simulink library "LopesDevelopmentLibrary"  (R2015b)
settings: Solver=ode45  StartTime=0.0  StopTime=10.0  RelTol=1e-3
values from neighbouring files (symbols this model uses):
  d2r = @(d) d*(pi/180)    [LopesDevelopmentLibrary_LoadParameters.m]
  ts = LopesParams.ts    [LopesDevelopmentLibrary_LoadParameters.m]
undefined symbols (not defined in the file or in its folder): anyParameterChanged, DiscIntNeverNeededParam, gcbh, LHF, LKF, LopesParams, macaddr, mxpcnetworkconfig, mxpcrtudprx, mxpcrtudptx, patientParametersChanged, port, PX, PZ, RHF, RKF, SelectorLOPESInSize, StrideTime_s, Time
undefined symbols (not defined in the file): LopesParamsSendDataArrayLen
libraries: LopesDevelopmentLibrary x288, simulink x98, dspmtrx3 x47, xpciplib x6, xpcnetworkbufferlib x5, dspsigops x4, dspstat3 x3, xpcethernetlib x2, visionstatistics x2, xpcseriallib x2, nmc x1, simulink_extras x1
(part 10 of 12)

== system LopesDevelopmentLibrary/Mindwalker/Mindwalker_Lopes_Conversion/VisualizeStickFigure/Subsystem ==
  In1 : Inport
  Enable : EnablePort
  Interpreted MATLAB Function : MATLABFcn  MATLABFcn=Mindwalker_ShowStickFigure  OutputDimensions=0
  wires:
  In1/1 -> Interpreted MATLAB Function/1

== system LopesDevelopmentLibrary/Robot control blocks/FromLopes/ParseString/MeasuredSegmentToAnatomicAngles ==
  note: This block works for angles, angular velocities and accelerations as well.
  note: Order of the signals:
      | PX (forward)
      | PZ (right)
      | LHA (Left hip abduction)
      | LHF (Left hip flexion)
      | LKF (Left knee flexion)
      | RHA
      | RHF
      | RKF
      |
      | PY (up)
      | PAX (Pelvis axial rotation (right hip forward=positive?)
      | POB (Pelvis obliquity (left hip up =positive)
  segmentModelX : Inport
  Demux3 : Demux  Outputs=15
  MinusRHA : UnaryMinus
  Mux : Mux  Inputs=11
  SubtractKLF : Sum  Inputs=+-
  SubtractRKF : Sum  Inputs=+-
  Terminator{1..4} (4 alike) : Terminator
  Anatomic : Outport
  wires:
  Demux3/14 -> Terminator2/1  "LAE"
  Demux3/13 -> Mux/11  "POB"
  Demux3/12 -> Mux/10  "PAX"
  Demux3/11 -> Mux/9  "PY"
  Demux3/15 -> Terminator1/1  "RAE"
  Mux/1 -> Anatomic/1
  Demux3/7 -> MinusRHA/1  "RHA"
  segmentModelX/1 -> Demux3/1
  SubtractRKF/1 -> Mux/8  "RKF"
  Demux3/8 -> Mux/7, SubtractRKF/1  "RHF"
  MinusRHA/1 -> Mux/6  "RHA"
  SubtractKLF/1 -> Mux/5  "LKF"
  Demux3/4 -> Mux/4, SubtractKLF/1  "LHF"
  Demux3/3 -> Mux/3  "LHA"
  Demux3/2 -> Mux/2  "PZ"
  Demux3/1 -> Mux/1  "PX"
  Demux3/5 -> SubtractKLF/2  "RHA"
  Demux3/6 -> Terminator4/1  "RHF"
  Demux3/9 -> SubtractRKF/2  "RHF"
  Demux3/10 -> Terminator3/1

== system LopesDevelopmentLibrary/Robot control blocks/FromLopes/ParseString/MeasuredSegmentToAnatomicAngles1 ==
  note: Order of the signals:
      | PX (forward)
      | PZ (right)
      | LHA (Left hip abduction)
      | LHF (Left hip flexion)
      | LKF (Left knee flexion)
      | RHA
      | RHF
      | RKF
      |
      | PY (up)
      | PAX (Pelvis axial rotation (right hip forward=positive?)
      | POB (Pelvis obliquity (left hip up =positive)
  note: This block works for angles, angular velocities and accelerations as well.
  segmentModelX : Inport
  Demux3 : Demux  Outputs=15
  MinusRHA : UnaryMinus
  Mux : Mux  Inputs=11
  SubtractKLF : Sum  Inputs=+-
  SubtractRKF : Sum  Inputs=+-
  Terminator{1..4} (4 alike) : Terminator
  Anatomic : Outport
  wires:
  Demux3/10 -> Terminator3/1
  Demux3/9 -> SubtractRKF/2  "RHF"
  Demux3/6 -> Terminator4/1  "RHF"
  Demux3/5 -> SubtractKLF/2  "RHA"
  Demux3/1 -> Mux/1  "PX"
  Demux3/2 -> Mux/2  "PZ"
  Demux3/3 -> Mux/3  "LHA"
  Demux3/4 -> SubtractKLF/1, Mux/4  "LHF"
  SubtractKLF/1 -> Mux/5  "LKF"
  MinusRHA/1 -> Mux/6  "RHA"
  Demux3/8 -> SubtractRKF/1, Mux/7  "RHF"
  SubtractRKF/1 -> Mux/8  "RKF"
  segmentModelX/1 -> Demux3/1
  Demux3/7 -> MinusRHA/1  "RHA"
  Mux/1 -> Anatomic/1
  Demux3/15 -> Terminator1/1  "RAE"
  Demux3/11 -> Mux/9  "PY"
  Demux3/12 -> Mux/10  "PAX"
  Demux3/13 -> Mux/11  "POB"
  Demux3/14 -> Terminator2/1  "LAE"

== system LopesDevelopmentLibrary/Robot control blocks/FromLopes/ParseString/MeasuredSegmentToAnatomicAngles2 ==
  note: This block works for angles, angular velocities and accelerations as well.
  note: Order of the signals:
      | PX (forward)
      | PZ (right)
      | LHA (Left hip abduction)
      | LHF (Left hip flexion)
      | LKF (Left knee flexion)
      | RHA
      | RHF
      | RKF
      |
      | PY (up)
      | PAX (Pelvis axial rotation (right hip forward=positive?)
      | POB (Pelvis obliquity (left hip up =positive)
  segmentModelX : Inport
  Demux3 : Demux  Outputs=15
  MinusRHA : UnaryMinus
  Mux : Mux  Inputs=11
  SubtractKLF : Sum  Inputs=+-
  SubtractRKF : Sum  Inputs=+-
  Terminator{1..4} (4 alike) : Terminator
  Anatomic : Outport
  wires:
  Demux3/14 -> Terminator2/1  "LAE"
  Demux3/13 -> Mux/11  "POB"
  Demux3/12 -> Mux/10  "PAX"
  Demux3/11 -> Mux/9  "PY"
  Demux3/15 -> Terminator1/1  "RAE"
  Mux/1 -> Anatomic/1
  Demux3/7 -> MinusRHA/1  "RHA"
  segmentModelX/1 -> Demux3/1
  SubtractRKF/1 -> Mux/8  "RKF"
  Demux3/8 -> Mux/7, SubtractRKF/1  "RHF"
  MinusRHA/1 -> Mux/6  "RHA"
  SubtractKLF/1 -> Mux/5  "LKF"
  Demux3/4 -> Mux/4, SubtractKLF/1  "LHF"
  Demux3/3 -> Mux/3  "LHA"
  Demux3/2 -> Mux/2  "PZ"
  Demux3/1 -> Mux/1  "PX"
  Demux3/5 -> SubtractKLF/2  "RHA"
  Demux3/6 -> Terminator4/1  "RHF"
  Demux3/9 -> SubtractRKF/2  "RHF"
  Demux3/10 -> Terminator3/1

== system LopesDevelopmentLibrary/Robot control blocks/FromLopes/ParseString/MeasuredSegmentToAnatomicAngles3 ==
  note: Order of the signals:
      | PX (forward)
      | PZ (right)
      | LHA (Left hip abduction)
      | LHF (Left hip flexion)
      | LKF (Left knee flexion)
      | RHA
      | RHF
      | RKF
      |
      | PY (up)
      | PAX (Pelvis axial rotation (right hip forward=positive?)
      | POB (Pelvis obliquity (left hip up =positive)
  note: This block works for angles, angular velocities and accelerations as well.
  segmentModelX : Inport
  Demux3 : Demux  Outputs=15
  MinusRHA : UnaryMinus
  Mux : Mux  Inputs=11
  SubtractKLF : Sum  Inputs=+-
  SubtractRKF : Sum  Inputs=+-
  Terminator{1..4} (4 alike) : Terminator
  Anatomic : Outport
  wires:
  Demux3/10 -> Terminator3/1
  Demux3/9 -> SubtractRKF/2  "RHF"
  Demux3/6 -> Terminator4/1  "RHF"
  Demux3/5 -> SubtractKLF/2  "RHA"
  Demux3/1 -> Mux/1  "PX"
  Demux3/2 -> Mux/2  "PZ"
  Demux3/3 -> Mux/3  "LHA"
  Demux3/4 -> SubtractKLF/1, Mux/4  "LHF"
  SubtractKLF/1 -> Mux/5  "LKF"
  MinusRHA/1 -> Mux/6  "RHA"
  Demux3/8 -> SubtractRKF/1, Mux/7  "RHF"
  SubtractRKF/1 -> Mux/8  "RKF"
  segmentModelX/1 -> Demux3/1
  Demux3/7 -> MinusRHA/1  "RHA"
  Mux/1 -> Anatomic/1
  Demux3/15 -> Terminator1/1  "RAE"
  Demux3/11 -> Mux/9  "PY"
  Demux3/12 -> Mux/10  "PAX"
  Demux3/13 -> Mux/11  "POB"
  Demux3/14 -> Terminator2/1  "LAE"

== system LopesDevelopmentLibrary/Robot control blocks/FromLopes/ParseString/MeasuredSegmentToAnatomicForce ==
  note: We can (at this moment) only get the joint forces of the patient
      | in absolute torques, i.e. torques on the limbs instead of joint torques. In order to
      | convert this to (relative) anatomical torques, we need this block.
      | This block works for forces/torques only (it does the inverse transformation
      | of the MeasuredSegmentToAnatomicVelocity block).
  segmentMeasForce : Inport
  AddLHF : Sum
  AddRHF : Sum
  Demux3 : Demux  Outputs=10
  MinusLKF : UnaryMinus
  MinusRHA : UnaryMinus
  MinusRKF : UnaryMinus
  Mux : Mux  Inputs=8
  Terminator : Terminator
  Terminator1 : Terminator
  AnatomicForce : Outport
  wires:
  Demux3/6 -> Terminator1/1  "RHF"
  Demux3/8 -> AddRHF/1  "RHF"
  Mux/1 -> AnatomicForce/1
  Demux3/7 -> MinusRHA/1  "RHA"
  MinusRKF/1 -> Mux/8  "RKF"
  AddRHF/1 -> Mux/7  "RHF"
  MinusRHA/1 -> Mux/6  "RHA"
  AddLHF/1 -> Mux/4  "LHF"
  Demux3/3 -> Mux/3  "LHA"
  Demux3/2 -> Mux/2  "PZ"
  Demux3/1 -> Mux/1  "PX"
  Demux3/9 -> AddRHF/2, MinusRKF/1  "RHF"
  Demux3/10 -> Terminator/1
  Demux3/4 -> AddLHF/1  "LHF"
  Demux3/5 -> AddLHF/2, MinusLKF/1  "RHA"
  MinusLKF/1 -> Mux/5  "LKF"
  segmentMeasForce/1 -> Demux3/1

== system LopesDevelopmentLibrary/Robot control blocks/FromLopes/ParseString/Vector2CartesianPositionsBus ==
  note: Output:
      | Cartesian positions (i.e., 3-element vectors) of:
      | Pelvis
      | LeftHip
      | LeftKnee
      | LeftAnkle
      | RightHip
      | RightKnee
      | RightAnkle
      |
      | Each vector: [X,Y, Z] = [Forward, Up, Right]
  In : Inport
  Demux3 : Demux  Outputs=11
  Mux : Mux  Inputs=7
  Terminator{1..4} (4 alike) : Terminator
  CartesianPositions : Outport
  wires:
  Demux3/9 -> Mux/7  "pRightAnkle"
  Demux3/4 -> Mux/4  "pLeftAnkle"
  Demux3/1 -> Mux/1  "pPelvis"
  Demux3/2 -> Mux/2  "pLeftHip"
  Demux3/3 -> Mux/3  "pLeftKnee"
  Demux3/5 -> Terminator1/1  "pLeftHeel"
  Demux3/6 -> Terminator4/1  "pLeftToe"
  Demux3/7 -> Mux/5  "pRightHip"
  Demux3/8 -> Mux/6  "pRightKnee"
  Demux3/10 -> Terminator2/1  "pRightHeel"
  Demux3/11 -> Terminator3/1  "pRightToe"
  In/1 -> Demux3/1
  Mux/1 -> CartesianPositions/1

== system LopesDevelopmentLibrary/Robot control blocks/FromLopes/ParseString/~Debug ==

== system LopesDevelopmentLibrary/Robot control blocks/ToLopes/GenerateVelocities/UseNumericalDerivative ==
  Positions : Inport
  Enable : EnablePort
  Discrete Derivative : simulink/Discrete/Discrete Derivative  gainval=1.0  ICPrevScaledInput=0.0  InputProcessing=Inherited  OutMin=[]  OutMax=[]  OutDataType=fixdt(1, 16)  OutScaling=2^-10  DoSatur=off
  Gain : Gain
  Velocities : Outport
  wires:
  Positions/1 -> Discrete Derivative/1
  Discrete Derivative/1 -> Gain/1
  Gain/1 -> Velocities/1

== system LopesDevelopmentLibrary/Robot control blocks/ToLopes/GenerateVelocities/UseNumericalDerivativeFiltered ==
  Positions : Inport
  Enable : EnablePort
  FirstOrderLowPassFilter : Subsystem  mask{Tau=0.01}
  Gain : Gain
  Velocities : Outport
  wires:
  FirstOrderLowPassFilter/1(ddt) -> Gain/1
  Positions/1 -> FirstOrderLowPassFilter/1(In)
  Gain/1 -> Velocities/1

== system LopesDevelopmentLibrary/Robot control blocks/ToLopes/GenerateVelocities/UseUserVelocity ==
  Velocities_in : Inport
  Enable : EnablePort
  Gain : Gain  Gain=ones(1,8)
  Velocities : Outport
  wires:
  Velocities_in/1 -> Gain/1
  Gain/1 -> Velocities/1

== system LopesDevelopmentLibrary/Robot control blocks/ToLopes/GenerateVelocities/UseZeros ==
  Enable : EnablePort
  Constant : Constant  Value=[0,0,0,0,0,0,0,0]
  Velocities : Outport  InitialOutput=[0,0,0,0,0,0,0,0]
  wires:
  Constant/1 -> Velocities/1

== system LopesDevelopmentLibrary/Robot control blocks/ToLopes/SwitchVelocitiesOnly/UseAnalyticalVelocityOnly ==
  ModelPosIn : Inport
  DesSprPos : Inport  Port=2
  DesSprVel : Inport  Port=3
  Enable : EnablePort
  Add : Sum  Inputs=-+
  Add1 : Sum
  Constant : Constant  Value=0  OutDataTypeStr=boolean
  Constant1 : Constant  Value=[0,0,0,0,0,0,0,0]
  OneOverTau_s : Gain
  UpdateSpringPos : Outport  InitialOutput=[false]
  SpringPositions : Outport  Port=2  InitialOutput=[0,0,0,0,0,0,0,0]
  SpringVelocities : Outport  Port=3  InitialOutput=[0,0,0,0,0,0,0,0]
  wires:
  Constant1/1 -> SpringPositions/1
  Constant/1 -> UpdateSpringPos/1
  Add1/1 -> SpringVelocities/1
  Add/1 -> OneOverTau_s/1
  OneOverTau_s/1 -> Add1/1
  DesSprVel/1 -> Add1/2
  DesSprPos/1 -> Add/2
  ModelPosIn/1 -> Add/1

== system LopesDevelopmentLibrary/Robot control blocks/ToLopes/SwitchVelocitiesOnly/UsePositionsAndVelocities ==
  DesSprPos : Inport
  DesSprVel : Inport  Port=2
  Enable : EnablePort
  Constant : Constant  Value=true  OutDataTypeStr=boolean
  UpdateSpringPos : Outport  InitialOutput=[false]
  SpringPositions : Outport  Port=2  InitialOutput=[0,0,0,0,0,0,0,0]
  SpringVelocities : Outport  Port=3  InitialOutput=[0,0,0,0,0,0,0,0]
  wires:
  Constant/1 -> UpdateSpringPos/1
  DesSprVel/1 -> SpringVelocities/1
  DesSprPos/1 -> SpringPositions/1

== system LopesDevelopmentLibrary/BlocksForInternalUse/LLC Communication/LLC Network Configuration/Variant Network Init/Init_NonRT_UDP ==
  note: No initialization needed for Non RT UDP.
  Dummy_in : Inport
  Dummy1 : Terminator
  Dummy2 : Constant
  Dummy_out : Outport
  wires:
  Dummy_in/1 -> Dummy1/1
  Dummy2/1 -> Dummy_out/1

== system LopesDevelopmentLibrary/BlocksForInternalUse/LLC Communication/LLC Network Configuration/Variant Network Init/Init_RT_2012b ==
  Dummy_in : Inport
  Dummy1 : Terminator
  Dummy2 : Constant
  "Network Configuration_RT_2012b " : LopesDevelopmentLibrary/BlocksForInternalUse/LLC Communication/UDP_Blocks/Network Configuration_RT_2012b   IpAddress=LopesParams.Communication.ipSelf_RT  SubnetMask=255.255.255.0  Gateway=0.0.0.0  EthDrv=Intel Gigabit  PciBus=LopesParams.Communication.busSelf_RT  PciSlot=LopesParams.Communication.slotSelf_RT
  Dummy_out : Outport
  wires:
  Dummy2/1 -> Dummy_out/1
  Dummy_in/1 -> Dummy1/1

== system LopesDevelopmentLibrary/BlocksForInternalUse/LLC Communication/LLC Network Configuration/Variant Network Init/Init_RT_2014b ==
  Dummy_in : Inport
  Dummy2 : Constant
  Dummy3 : Terminator
  "Network Configuration_RT_2014b " : LopesDevelopmentLibrary/BlocksForInternalUse/LLC Communication/UDP_Blocks/Network Configuration_RT_2014b   ID=1  IpAddress=LopesParams.Communication.ipSelf_RT  SubnetMask=255.255.255.0  Gateway=0.0.0.0  EthDrv=Intel Gigabit  PciBus=LopesParams.Communication.busSelf_RT  PciSlot=LopesParams.Communication.slotSelf_RT  udpID=0
  Dummy_out : Outport
  wires:
  Dummy_in/1 -> Dummy3/1
  Dummy2/1 -> Dummy_out/1

== system LopesDevelopmentLibrary/BlocksForInternalUse/LLC Communication/LLC Network Configuration/Variant Network Init/Init_RT_2015b ==
  Dummy_in : Inport
  Dummy2 : Constant
  Dummy3 : Terminator
  Network Configuration_RT_2015b : LopesDevelopmentLibrary/BlocksForInternalUse/LLC Communication/UDP_Blocks/Network Configuration_RT_2015b  ID=1  IpAddress=LopesParams.Communication.ipSelf_RT  SubnetMask=255.255.255.0  Gateway=0.0.0.0  EthDrv=Intel Gigabit  PciBus=LopesParams.Communication.busSelf_RT  PciSlot=LopesParams.Communication.slotSelf_RT  udpID=0  MulticastList=[]  Multicast={}
  Dummy_out : Outport
  wires:
  Dummy2/1 -> Dummy_out/1
  Dummy_in/1 -> Dummy3/1

== system LopesDevelopmentLibrary/BlocksForInternalUse/LLC Communication/LLCReceiveUDP/UDPReceiveVariantChannel/Receive_Non_RT ==
  Dummy_in : Inport
  Receive_Non-RT : LopesDevelopmentLibrary/BlocksForInternalUse/LLC Communication/UDP_Blocks/Receive_Non-RT  ipAddress='0.0.0.0'  ipPort=port  width=1500  vblLen=on  sampletime=LopesParams.ts
  Terminator : Terminator
  RecvData : Outport
  RecvLen : Outport  Port=2
  wires:
  Receive_Non-RT/2 -> RecvLen/1
  Receive_Non-RT/1 -> RecvData/1
  Dummy_in/1 -> Terminator/1

== system LopesDevelopmentLibrary/BlocksForInternalUse/LLC Communication/LLCReceiveUDP/UDPReceiveVariantChannel/Receive_RT_2015b ==
  Dummy_in : Inport
  Receive_RT_2015b : LopesDevelopmentLibrary/BlocksForInternalUse/LLC Communication/UDP_Blocks/Receive_RT_2015b  ID=1  Receive1='0.0.0.0'  Receive2=port  Receive3=1500  Receive4=LopesParams.ts  udpID=0
  Terminator : Terminator
  RecvData : Outport
  RecvLen : Outport  Port=2
  wires:
  Dummy_in/1 -> Terminator/1
  Receive_RT_2015b/1 -> RecvData/1
  Receive_RT_2015b/2 -> RecvLen/1

== system LopesDevelopmentLibrary/BlocksForInternalUse/LLC Communication/LLCReceiveUDP/UDPReceiveVariantChannel/Receive_RT_R2012b ==
  Dummy_in : Inport
  "Receive_RT_2012b " : LopesDevelopmentLibrary/BlocksForInternalUse/LLC Communication/UDP_Blocks/Receive_RT_2012b   Receive1='0.0.0.0'  Receive2=port  Receive3=1500  Receive4=LopesParams.ts
  Terminator : Terminator
  RecvData : Outport
  RecvLen : Outport  Port=2
  wires:
  "Receive_RT_2012b "/1 -> RecvData/1
  "Receive_RT_2012b "/2 -> RecvLen/1
  Dummy_in/1 -> Terminator/1

== system LopesDevelopmentLibrary/BlocksForInternalUse/LLC Communication/LLCReceiveUDP/UDPReceiveVariantChannel/Receive_RT_R2014b ==
  Dummy_in : Inport
  "Receive_RT_2014b " : LopesDevelopmentLibrary/BlocksForInternalUse/LLC Communication/UDP_Blocks/Receive_RT_2014b   ID=1  Receive1='0.0.0.0'  Receive2=port  Receive3=1500  Receive4=LopesParams.ts  udpID=0
  Terminator : Terminator
  RecvData : Outport
  RecvLen : Outport  Port=2
  wires:
  "Receive_RT_2014b "/2 -> RecvLen/1
  "Receive_RT_2014b "/1 -> RecvData/1
  Dummy_in/1 -> Terminator/1

== system LopesDevelopmentLibrary/BlocksForInternalUse/LLC Communication/LLCSendUDP/UDPSendVariant/UDPSendVariantChannel ==
  note: 1) Add Subsystem or Model blocks as valid variant choices.
      | 2) You cannot connect blocks at this level. At simulation, connectivity is automatically
      | determined, based on the active variant and port name matching.
  SendData : Inport
  SendLen : Inport  Port=2
  Send_Non_RT : Subsystem  VariantControl=LopesVariant_Non_RT
  Send_RT_2012b : Subsystem  VariantControl=LopesVariant_RT_2012b
  Send_RT_2014b : Subsystem  VariantControl=LopesVariant_RT_2014b
  Send_RT_2015b : Subsystem  VariantControl=LopesVariant_RT_2015b
  Dummy_out : Outport

== system LopesDevelopmentLibrary/GaitGeneration/CalculateBreaksCoefs/Calculate/PelvisTZ1/AdjustAmplitude ==
  note: This block multiplies all positions, velocities and accelerations of the first 3 key Events by input V_left,
      | and the last 3 key Events by V_right. In other words,  it just scales the amplitude of the part of the curve for
      | weight shift left and right.
  M : Inport
  V_left : Inport  Port=2
  V_right : Inport  Port=3
  Matrix Concatenate : Concatenate  Mode=Multidimensional array  ConcatenateDimension=2
  Matrix Concatenate1 : Concatenate  Mode=Multidimensional array
  Product : Product  RndMeth=Zero
  Product1 : Product  RndMeth=Zero
  angle_vel_accLeft : dspmtrx3/Submatrix  RowSpan=Range of rows  RowStartMode=First  RowStartIndex=1  RowEndMode=Index  RowEndIndex=3  ColSpan=Range of columns  ColStartMode=Index  ColStartIndex=2  ColEndMode=Last  ColEndIndex=1
  angle_vel_accRight : dspmtrx3/Submatrix  RowSpan=Range of rows  RowStartMode=Index  RowStartIndex=4  RowEndMode=Last  RowEndIndex=3  ColSpan=Range of columns  ColStartMode=Index  ColStartIndex=2  ColEndMode=Last  ColEndIndex=1
  times : dspmtrx3/Submatrix  RowSpan=All rows  RowStartMode=First  RowStartIndex=1  RowEndMode=Last  RowEndIndex=1  ColSpan=One column  ColStartMode=First  ColStartIndex=1  ColEndMode=Last  ColEndIndex=1
  Y : Outport
  wires:
  V_left/1 -> Product/2
  M/1 -> angle_vel_accRight/1, angle_vel_accLeft/1, times/1
  Matrix Concatenate/1 -> Y/1
  angle_vel_accLeft/1 -> Product/1
  times/1 -> Matrix Concatenate/1
  Product/1 -> Matrix Concatenate1/1
  angle_vel_accRight/1 -> Product1/1
  V_right/1 -> Product1/2
  Product1/1 -> Matrix Concatenate1/2
  Matrix Concatenate1/1 -> Matrix Concatenate/2

== system LopesDevelopmentLibrary/GaitGeneration/CalculateBreaksCoefs/Calculate/PelvisTZ1/AdjustDurationLeft ==
  note: This block makes the weight shift from one leg to the other leg
      | faster (not slower, that would immediately lead to a key event order exception).
      | It does this by shifting the 'extreme' key event (number 2 for durationLeft,
      | no 5 for durationRight) an amount of V earlier, and the 'midpoint' key event
      | (number 1 resp. 4) an amount of V/2 earlier.
      | The velocity and accelearation of the midpoint key event need to
      | be compensated accordingly:
      |
      | v_new = v_old * deltaT_old/deltaT_new,
      | where deltaT is the time between the extreme key events
      |  (KE2-KE6 for left, KE5-KE3 for right).
  M : Inport
  V : Inport  Port=2
  DeltaT_new : Sum  Inputs=+-
  DeltaT_old : Sum  Inputs=+-
  Demux : Demux  Outputs=2
  Demux1 : Demux  Outputs=2
  Divide : Product  Inputs=*/
  Gain : Gain  Gain=0.5
  GetRelevantTimesForDeltaTCalculation : Selector  NumberOfDimensions=2  InputPortWidth=3  IndexOptions=Index vector (dialog),Index vector (dialog)  Indices=[keyEventsToAffect(2) keyEventBeforeAffected],1  OutputSizes=1,1
  GetRelevantTimesForDeltaTCalculation1 : Selector  NumberOfDimensions=2  InputPortWidth=3  IndexOptions=Index vector (dialog),Index vector (dialog)  Indices=[keyEventsToAffect(2) keyEventBeforeAffected],1  OutputSizes=1,1
  PhaseWrapper : LopesDevelopmentLibrary/Various/PhaseWrapper
  PhaseWrapper1 : LopesDevelopmentLibrary/Various/PhaseWrapper
  adjustTimingKE1 : LopesDevelopmentLibrary/Various/AddToMatrixElement  row=keyEventsToAffect(1)  col=1  minimum=-inf  maximum=inf
  adjustTimingKE2 : LopesDevelopmentLibrary/Various/AddToMatrixElement  row=keyEventsToAffect(2)  col=1  minimum=-inf  maximum=inf
  adjustVelocityKE1 : LopesDevelopmentLibrary/Various/MultiplyMatrixElement  row=keyEventsToAffect(1)  col=3  minimum=-inf  maximum=inf
  Y : Outport
  wires:
  PhaseWrapper1/1 -> Divide/2
  GetRelevantTimesForDeltaTCalculation1/1 -> Demux1/1
  PhaseWrapper/1 -> Divide/1
  adjustVelocityKE1/1 -> Y/1
  Divide/1 -> adjustVelocityKE1/2
  DeltaT_new/1 -> PhaseWrapper1/1
  DeltaT_old/1 -> PhaseWrapper/1
  Demux1/2 -> DeltaT_new/2  "T_start"
  Demux1/1 -> DeltaT_new/1  "T_end"
  adjustTimingKE2/1 -> adjustVelocityKE1/1, GetRelevantTimesForDeltaTCalculation1/1
  Demux/2 -> DeltaT_old/2  "T_start"
  Demux/1 -> DeltaT_old/1  "T_end"
  GetRelevantTimesForDeltaTCalculation/1 -> Demux/1
  Gain/1 -> adjustTimingKE1/2
  M/1 -> adjustTimingKE1/1, GetRelevantTimesForDeltaTCalculation/1
  V/1 -> adjustTimingKE2/2, Gain/1
  adjustTimingKE1/1 -> adjustTimingKE2/1

== system LopesDevelopmentLibrary/GaitGeneration/CalculateBreaksCoefs/Calculate/PelvisTZ1/AdjustDurationRight ==
  note: This block makes the weight shift from one leg to the other leg
      | faster (not slower, that would immediately lead to a key event order exception).
      | It does this by shifting the 'extreme' key event (number 2 for durationLeft,
      | no 5 for durationRight) an amount of V earlier, and the 'midpoint' key event
      | (number 1 resp. 4) an amount of V/2 earlier.
      | The velocity and accelearation of the midpoint key event need to
      | be compensated accordingly:
      |
      | v_new = v_old * deltaT_old/deltaT_new,
      | where deltaT is the time between the extreme key events
      |  (KE2-KE6 for left, KE5-KE3 for right).
  M : Inport
  V : Inport  Port=2
  DeltaT_new : Sum  Inputs=+-
  DeltaT_old : Sum  Inputs=+-
  Demux : Demux  Outputs=2
  Demux1 : Demux  Outputs=2
  Divide : Product  Inputs=*/
  Gain : Gain  Gain=0.5
  GetRelevantTimesForDeltaTCalculation : Selector  NumberOfDimensions=2  InputPortWidth=3  IndexOptions=Index vector (dialog),Index vector (dialog)  Indices=[keyEventsToAffect(2) keyEventBeforeAffected],1  OutputSizes=1,1
  GetRelevantTimesForDeltaTCalculation1 : Selector  NumberOfDimensions=2  InputPortWidth=3  IndexOptions=Index vector (dialog),Index vector (dialog)  Indices=[keyEventsToAffect(2) keyEventBeforeAffected],1  OutputSizes=1,1
  PhaseWrapper : LopesDevelopmentLibrary/Various/PhaseWrapper
  PhaseWrapper1 : LopesDevelopmentLibrary/Various/PhaseWrapper
  adjustTimingKE1 : LopesDevelopmentLibrary/Various/AddToMatrixElement  row=keyEventsToAffect(1)  col=1  minimum=-inf  maximum=inf
  adjustTimingKE2 : LopesDevelopmentLibrary/Various/AddToMatrixElement  row=keyEventsToAffect(2)  col=1  minimum=-inf  maximum=inf
  adjustVelocityKE1 : LopesDevelopmentLibrary/Various/MultiplyMatrixElement  row=keyEventsToAffect(1)  col=3  minimum=-inf  maximum=inf
  Y : Outport
  wires:
  PhaseWrapper1/1 -> Divide/2
  GetRelevantTimesForDeltaTCalculation1/1 -> Demux1/1
  PhaseWrapper/1 -> Divide/1
  adjustVelocityKE1/1 -> Y/1
  Divide/1 -> adjustVelocityKE1/2
  DeltaT_new/1 -> PhaseWrapper1/1
  DeltaT_old/1 -> PhaseWrapper/1
  Demux1/2 -> DeltaT_new/2  "T_start"
  Demux1/1 -> DeltaT_new/1  "T_end"
  adjustTimingKE2/1 -> adjustVelocityKE1/1, GetRelevantTimesForDeltaTCalculation1/1
  Demux/2 -> DeltaT_old/2  "T_start"
  Demux/1 -> DeltaT_old/1  "T_end"
  GetRelevantTimesForDeltaTCalculation/1 -> Demux/1
  Gain/1 -> adjustTimingKE1/2
  M/1 -> adjustTimingKE1/1, GetRelevantTimesForDeltaTCalculation/1
  V/1 -> adjustTimingKE2/2, Gain/1
  adjustTimingKE1/1 -> adjustTimingKE2/1

== system LopesDevelopmentLibrary/GaitGeneration/CalculateBreaksCoefs/Calculate/Time1/CalculateStrideLength ==
  note: This block calculates the step length: It calculates the positions of the left and right ankle
      | during stance phase, at 5 and 55 % of the gait cycle (we need both to accomodate for
      | a-symmetric gaits) and takes the difference in x position of both ankles. These are the
      | left and right step length. The sum of these is the stride length.
      | This block can be optimized computationally. However, in order to keep the number of
      | different library blocks small, I decided to first see if we'll easily make it in the computational
      | sense.
  BreaksCoefsBus : Inport
  Parameters : Inport  Port=2
  Add : Sum
  GenerateReferencePoseLeftFront : Subsystem
  GenerateReferencePoseRightFront : Subsystem
  LeftHeelX : Selector  InputPortWidth=21  IndexOptions=Index vector (dialog)  Indices=[10]  OutputSizes=1
  LeftHeelX1 : Selector  InputPortWidth=21  IndexOptions=Index vector (dialog)  Indices=[10]  OutputSizes=1
  PctDoublesupport LeftFront : Constant  Value=5
  PctDoublesupport RightFront : Constant  Value=55
  RightHeelX : Selector  InputPortWidth=21  IndexOptions=Index vector (dialog)  Indices=[19]  OutputSizes=1
  RightHeelX1 : Selector  InputPortWidth=21  IndexOptions=Index vector (dialog)  Indices=[19]  OutputSizes=1
  Subtract : Sum  Inputs=+-
  Subtract1 : Sum  Inputs=-+
  StrideLength : Outport
  wires:
  Parameters/1 -> GenerateReferencePoseRightFront/3(Parameters), GenerateReferencePoseLeftFront/3(Parameters)
  PctDoublesupport LeftFront/1 -> GenerateReferencePoseLeftFront/1(Phase)
  BreaksCoefsBus/1 -> GenerateReferencePoseRightFront/2(BreaksCoefs), GenerateReferencePoseLeftFront/2(BreaksCoefs)
  LeftHeelX/1 -> Subtract/1
  RightHeelX/1 -> Subtract/2
  Subtract/1 -> Add/1
  Add/1 -> StrideLength/1
  LeftHeelX1/1 -> Subtract1/1
  RightHeelX1/1 -> Subtract1/2
  PctDoublesupport RightFront/1 -> GenerateReferencePoseRightFront/1(Phase)
  Subtract1/1 -> Add/2
  GenerateReferencePoseLeftFront/1(CartesianPositions) -> LeftHeelX/1, RightHeelX/1
  GenerateReferencePoseRightFront/1(CartesianPositions) -> RightHeelX1/1, LeftHeelX1/1

== system LopesDevelopmentLibrary/GaitGenerationExtra/CalculateBreaksCoefs/Calculate/PelvisTZ1/AdjustAmplitude ==
  note: This block multiplies all positions, velocities and accelerations of the first 3 key Events by input V_left,
      | and the last 3 key Events by V_right. In other words,  it just scales the amplitude of the part of the curve for
      | weight shift left and right.
  M : Inport
  V_left : Inport  Port=2
  V_right : Inport  Port=3
  Matrix Concatenate : Concatenate  Mode=Multidimensional array  ConcatenateDimension=2
  Matrix Concatenate1 : Concatenate  Mode=Multidimensional array
  Product : Product  RndMeth=Zero
  Product1 : Product  RndMeth=Zero
  angle_vel_accLeft : dspmtrx3/Submatrix  RowSpan=Range of rows  RowStartMode=First  RowStartIndex=1  RowEndMode=Index  RowEndIndex=3  ColSpan=Range of columns  ColStartMode=Index  ColStartIndex=2  ColEndMode=Last  ColEndIndex=1
  angle_vel_accRight : dspmtrx3/Submatrix  RowSpan=Range of rows  RowStartMode=Index  RowStartIndex=4  RowEndMode=Last  RowEndIndex=3  ColSpan=Range of columns  ColStartMode=Index  ColStartIndex=2  ColEndMode=Last  ColEndIndex=1
  times : dspmtrx3/Submatrix  RowSpan=All rows  RowStartMode=First  RowStartIndex=1  RowEndMode=Last  RowEndIndex=1  ColSpan=One column  ColStartMode=First  ColStartIndex=1  ColEndMode=Last  ColEndIndex=1
  Y : Outport
  wires:
  V_left/1 -> Product/2
  M/1 -> angle_vel_accRight/1, angle_vel_accLeft/1, times/1
  Matrix Concatenate/1 -> Y/1
  angle_vel_accLeft/1 -> Product/1
  times/1 -> Matrix Concatenate/1
  Product/1 -> Matrix Concatenate1/1
  angle_vel_accRight/1 -> Product1/1
  V_right/1 -> Product1/2
  Product1/1 -> Matrix Concatenate1/2
  Matrix Concatenate1/1 -> Matrix Concatenate/2

== system LopesDevelopmentLibrary/GaitGenerationExtra/CalculateBreaksCoefs/Calculate/PelvisTZ1/AdjustDurationLeft ==
  note: This block makes the weight shift from one leg to the other leg
      | faster (not slower, that would immediately lead to a key event order exception).
      | It does this by shifting the 'extreme' key event (number 2 for durationLeft,
      | no 5 for durationRight) an amount of V earlier, and the 'midpoint' key event
      | (number 1 resp. 4) an amount of V/2 earlier.
      | The velocity and accelearation of the midpoint key event need to
      | be compensated accordingly:
      |
      | v_new = v_old * deltaT_old/deltaT_new,
      | where deltaT is the time between the extreme key events
      |  (KE2-KE6 for left, KE5-KE3 for right).
  M : Inport
  V : Inport  Port=2
  DeltaT_new : Sum  Inputs=+-
  DeltaT_old : Sum  Inputs=+-
  Demux : Demux  Outputs=2
  Demux1 : Demux  Outputs=2
  Divide : Product  Inputs=*/
  Gain : Gain  Gain=0.5
  GetRelevantTimesForDeltaTCalculation : Selector  NumberOfDimensions=2  InputPortWidth=3  IndexOptions=Index vector (dialog),Index vector (dialog)  Indices=[keyEventsToAffect(2) keyEventBeforeAffected],1  OutputSizes=1,1
  GetRelevantTimesForDeltaTCalculation1 : Selector  NumberOfDimensions=2  InputPortWidth=3  IndexOptions=Index vector (dialog),Index vector (dialog)  Indices=[keyEventsToAffect(2) keyEventBeforeAffected],1  OutputSizes=1,1
  PhaseWrapper : LopesDevelopmentLibrary/Various/PhaseWrapper
  PhaseWrapper1 : LopesDevelopmentLibrary/Various/PhaseWrapper
  adjustTimingKE1 : LopesDevelopmentLibrary/Various/AddToMatrixElement  row=keyEventsToAffect(1)  col=1  minimum=-inf  maximum=inf
  adjustTimingKE2 : LopesDevelopmentLibrary/Various/AddToMatrixElement  row=keyEventsToAffect(2)  col=1  minimum=-inf  maximum=inf
  adjustVelocityKE1 : LopesDevelopmentLibrary/Various/MultiplyMatrixElement  row=keyEventsToAffect(1)  col=3  minimum=-inf  maximum=inf
  Y : Outport
  wires:
  PhaseWrapper1/1 -> Divide/2
  GetRelevantTimesForDeltaTCalculation1/1 -> Demux1/1
  PhaseWrapper/1 -> Divide/1
  adjustVelocityKE1/1 -> Y/1
  Divide/1 -> adjustVelocityKE1/2
  DeltaT_new/1 -> PhaseWrapper1/1
  DeltaT_old/1 -> PhaseWrapper/1
  Demux1/2 -> DeltaT_new/2  "T_start"
  Demux1/1 -> DeltaT_new/1  "T_end"
  adjustTimingKE2/1 -> adjustVelocityKE1/1, GetRelevantTimesForDeltaTCalculation1/1
  Demux/2 -> DeltaT_old/2  "T_start"
  Demux/1 -> DeltaT_old/1  "T_end"
  GetRelevantTimesForDeltaTCalculation/1 -> Demux/1
  Gain/1 -> adjustTimingKE1/2
  M/1 -> adjustTimingKE1/1, GetRelevantTimesForDeltaTCalculation/1
  V/1 -> adjustTimingKE2/2, Gain/1
  adjustTimingKE1/1 -> adjustTimingKE2/1

== system LopesDevelopmentLibrary/GaitGenerationExtra/CalculateBreaksCoefs/Calculate/PelvisTZ1/AdjustDurationRight ==
  note: This block makes the weight shift from one leg to the other leg
      | faster (not slower, that would immediately lead to a key event order exception).
      | It does this by shifting the 'extreme' key event (number 2 for durationLeft,
      | no 5 for durationRight) an amount of V earlier, and the 'midpoint' key event
      | (number 1 resp. 4) an amount of V/2 earlier.
      | The velocity and accelearation of the midpoint key event need to
      | be compensated accordingly:
      |
      | v_new = v_old * deltaT_old/deltaT_new,
      | where deltaT is the time between the extreme key events
      |  (KE2-KE6 for left, KE5-KE3 for right).
  M : Inport
  V : Inport  Port=2
  DeltaT_new : Sum  Inputs=+-
  DeltaT_old : Sum  Inputs=+-
  Demux : Demux  Outputs=2
  Demux1 : Demux  Outputs=2
  Divide : Product  Inputs=*/
  Gain : Gain  Gain=0.5
  GetRelevantTimesForDeltaTCalculation : Selector  NumberOfDimensions=2  InputPortWidth=3  IndexOptions=Index vector (dialog),Index vector (dialog)  Indices=[keyEventsToAffect(2) keyEventBeforeAffected],1  OutputSizes=1,1
  GetRelevantTimesForDeltaTCalculation1 : Selector  NumberOfDimensions=2  InputPortWidth=3  IndexOptions=Index vector (dialog),Index vector (dialog)  Indices=[keyEventsToAffect(2) keyEventBeforeAffected],1  OutputSizes=1,1
  PhaseWrapper : LopesDevelopmentLibrary/Various/PhaseWrapper
  PhaseWrapper1 : LopesDevelopmentLibrary/Various/PhaseWrapper
  adjustTimingKE1 : LopesDevelopmentLibrary/Various/AddToMatrixElement  row=keyEventsToAffect(1)  col=1  minimum=-inf  maximum=inf
  adjustTimingKE2 : LopesDevelopmentLibrary/Various/AddToMatrixElement  row=keyEventsToAffect(2)  col=1  minimum=-inf  maximum=inf
  adjustVelocityKE1 : LopesDevelopmentLibrary/Various/MultiplyMatrixElement  row=keyEventsToAffect(1)  col=3  minimum=-inf  maximum=inf
  Y : Outport
  wires:
  PhaseWrapper1/1 -> Divide/2
  GetRelevantTimesForDeltaTCalculation1/1 -> Demux1/1
  PhaseWrapper/1 -> Divide/1
  adjustVelocityKE1/1 -> Y/1
  Divide/1 -> adjustVelocityKE1/2
  DeltaT_new/1 -> PhaseWrapper1/1
  DeltaT_old/1 -> PhaseWrapper/1
  Demux1/2 -> DeltaT_new/2  "T_start"
  Demux1/1 -> DeltaT_new/1  "T_end"
  adjustTimingKE2/1 -> adjustVelocityKE1/1, GetRelevantTimesForDeltaTCalculation1/1
  Demux/2 -> DeltaT_old/2  "T_start"
  Demux/1 -> DeltaT_old/1  "T_end"
  GetRelevantTimesForDeltaTCalculation/1 -> Demux/1
  Gain/1 -> adjustTimingKE1/2
  M/1 -> adjustTimingKE1/1, GetRelevantTimesForDeltaTCalculation/1
  V/1 -> adjustTimingKE2/2, Gain/1
  adjustTimingKE1/1 -> adjustTimingKE2/1

== system LopesDevelopmentLibrary/GaitGenerationExtra/CalculateBreaksCoefs/Calculate/Time1/CalculateStrideLength ==
  note: This block calculates the step length: It calculates the positions of the left and right ankle
      | during stance phase, at 5 and 55 % of the gait cycle (we need both to accomodate for
      | a-symmetric gaits) and takes the difference in x position of both ankles. These are the
      | left and right step length. The sum of these is the stride length.
      | This block can be optimized computationally. However, in order to keep the number of
      | different library blocks small, I decided to first see if we'll easily make it in the computational
      | sense.
  BreaksCoefsBus : Inport
  Parameters : Inport  Port=2
  Add : Sum
  GenerateReferencePoseLeftFront : Subsystem
  GenerateReferencePoseRightFront : Subsystem
  LeftHeelX : Selector  InputPortWidth=21  IndexOptions=Index vector (dialog)  Indices=[10]  OutputSizes=1
  LeftHeelX1 : Selector  InputPortWidth=21  IndexOptions=Index vector (dialog)  Indices=[10]  OutputSizes=1
  PctDoublesupport LeftFront : Constant  Value=5
  PctDoublesupport RightFront : Constant  Value=55
  RightHeelX : Selector  InputPortWidth=21  IndexOptions=Index vector (dialog)  Indices=[19]  OutputSizes=1
  RightHeelX1 : Selector  InputPortWidth=21  IndexOptions=Index vector (dialog)  Indices=[19]  OutputSizes=1
  Subtract : Sum  Inputs=+-
  Subtract1 : Sum  Inputs=-+
  StrideLength : Outport
  wires:
  Parameters/1 -> GenerateReferencePoseRightFront/3(Parameters), GenerateReferencePoseLeftFront/3(Parameters)
  PctDoublesupport LeftFront/1 -> GenerateReferencePoseLeftFront/1(Phase)
  BreaksCoefsBus/1 -> GenerateReferencePoseRightFront/2(BreaksCoefs), GenerateReferencePoseLeftFront/2(BreaksCoefs)
  LeftHeelX/1 -> Subtract/1
  RightHeelX/1 -> Subtract/2
  Subtract/1 -> Add/1
  Add/1 -> StrideLength/1
  LeftHeelX1/1 -> Subtract1/1
  RightHeelX1/1 -> Subtract1/2
  PctDoublesupport RightFront/1 -> GenerateReferencePoseRightFront/1(Phase)
  Subtract1/1 -> Add/2
  GenerateReferencePoseLeftFront/1(CartesianPositions) -> LeftHeelX/1, RightHeelX/1
  GenerateReferencePoseRightFront/1(CartesianPositions) -> RightHeelX1/1, LeftHeelX1/1

== system LopesDevelopmentLibrary/GaitPhaseDetection/Gait Phase detection/LeftLeg/Heel strike_safety/Mean ==
  In1 : Inport
  Divide : Product  Inputs=*/
  Sum of Elements : Sum  Inputs=+
  Width : Width
  Out1 : Outport
  wires:
  Divide/1 -> Out1/1
  Sum of Elements/1 -> Divide/1
  Width/1 -> Divide/2
  In1/1 -> Sum of Elements/1, Width/1

== system LopesDevelopmentLibrary/GaitPhaseDetection/Gait Phase detection/RightLeg/Heel strike_safety1/Mean ==
  In1 : Inport
  Divide : Product  Inputs=*/
  Sum of Elements : Sum  Inputs=+
  Width : Width
  Out1 : Outport
  wires:
  Divide/1 -> Out1/1
  Sum of Elements/1 -> Divide/1
  Width/1 -> Divide/2
  In1/1 -> Sum of Elements/1, Width/1

== system LopesDevelopmentLibrary/Mindwalker/Mindwalker_Lopes_Conversion/TorsoDynamics/EndStops/CalculateDampingTerm ==
  note: Stiffness may be a vector.
  note: If stiffness is a vector,
      | Inertia may be a vector (but scalar is okay too)
  Stiffness : Inport
  Inertia : Inport  Port=2
  DampingCoef : Constant  Value=0.707
  Divide1 : Product  Inputs=*/
  OverrideInertia : Constant  Value=0
  Product1 : Product  Inputs=3  RndMeth=Zero
  Sqrt : Sqrt  SaturateOnIntegerOverflow=on
  Switch : Switch  Criteria=u2 ~= 0
  Two : Constant  Value=2
  Damping : Outport
  wires:
  Switch/1 -> Divide1/2
  OverrideInertia/1 -> Switch/1, Switch/2
  DampingCoef/1 -> Product1/1
  Two/1 -> Product1/2
  Sqrt/1 -> Product1/3
  Divide1/1 -> Sqrt/1
  Stiffness/1 -> Divide1/1
  Inertia/1 -> Switch/3
  Product1/1 -> Damping/1

== system LopesDevelopmentLibrary/Mindwalker/Mindwalker_Lopes_Conversion/TorsoDynamics/TorsoSpring/CalculateDampingTerm ==
  note: If stiffness is a vector,
      | Inertia may be a vector (but scalar is okay too)
  note: Stiffness may be a vector.
  Stiffness : Inport
  Inertia : Inport  Port=2
  DampingCoef : Constant  Value=0.707
  Divide1 : Product  Inputs=*/
  OverrideInertia : Constant  Value=1.5
  Product1 : Product  Inputs=3  RndMeth=Zero
  Sqrt : Sqrt  SaturateOnIntegerOverflow=on
  Switch : Switch  Criteria=u2 ~= 0
  Two : Constant  Value=2
  Damping : Outport
  wires:
  Product1/1 -> Damping/1
  Inertia/1 -> Switch/3
  Stiffness/1 -> Divide1/1
  Divide1/1 -> Sqrt/1
  Sqrt/1 -> Product1/3
  Two/1 -> Product1/2
  DampingCoef/1 -> Product1/1
  OverrideInertia/1 -> Switch/2, Switch/1
  Switch/1 -> Divide1/2

== system LopesDevelopmentLibrary/Robot control blocks/ToLopes/GenerateVelocities/UseNumericalDerivativeFiltered/FirstOrderLowPassFilter ==
  In : Inport
  Discrete-Time Integrator : DiscreteIntegrator  SampleTime=ts  ICPrevOutput=DiscIntNeverNeededParam  ICPrevScaledInput=DiscIntNeverNeededParam
  OneOverTau : Gain  Gain=1/Tau
  Sum : Sum  Inputs=|+-
  ddt : Outport
  wires:
  OneOverTau/1 -> Discrete-Time Integrator/1, ddt/1
  In/1 -> Sum/1
  Discrete-Time Integrator/1 -> Sum/2
  Sum/1 -> OneOverTau/1

== system LopesDevelopmentLibrary/BlocksForInternalUse/LLC Communication/LLCSendUDP/UDPSendVariant/UDPSendVariantChannel/Send_Non_RT ==
  SendData : Inport
  SendLen : Inport  Port=2
  Ground : Ground
  Send_Non-RT : LopesDevelopmentLibrary/BlocksForInternalUse/LLC Communication/UDP_Blocks/Send_Non-RT  ipAddress=LopesParams.Communication.ipLLC_NonRT  ipPort=port  localPort=-1  vblLen=on  sampletime=LopesParams.ts
  Dummy_out : Outport
  wires:
  SendData/1 -> Send_Non-RT/1
  SendLen/1 -> Send_Non-RT/2
  Ground/1 -> Dummy_out/1

== system LopesDevelopmentLibrary/BlocksForInternalUse/LLC Communication/LLCSendUDP/UDPSendVariant/UDPSendVariantChannel/Send_RT_2012b ==
  SendData : Inport
  SendLen : Inport  Port=2
  Ground : Ground
  Send_RT_2012b : LopesDevelopmentLibrary/BlocksForInternalUse/LLC Communication/UDP_Blocks/Send_RT_2012b  Send1=LopesParams.Communication.ipLLC_RT  Send2=port  Send3=-1  Send4=LopesParams.ts
  Dummy_out : Outport
  wires:
  SendData/1 -> Send_RT_2012b/1
  SendLen/1 -> Send_RT_2012b/2
  Ground/1 -> Dummy_out/1

== system LopesDevelopmentLibrary/BlocksForInternalUse/LLC Communication/LLCSendUDP/UDPSendVariant/UDPSendVariantChannel/Send_RT_2014b ==
  SendData : Inport
  SendLen : Inport  Port=2
  Ground : Ground
  Send_RT_2014b : LopesDevelopmentLibrary/BlocksForInternalUse/LLC Communication/UDP_Blocks/Send_RT_2014b  ID=1  Send1=LopesParams.Communication.ipLLC_RT  Send2=port  Send3=-1  Send4=LopesParams.ts  udpID=0
  Dummy_out : Outport
  wires:
  SendLen/1 -> Send_RT_2014b/2
  SendData/1 -> Send_RT_2014b/1
  Ground/1 -> Dummy_out/1

== system LopesDevelopmentLibrary/BlocksForInternalUse/LLC Communication/LLCSendUDP/UDPSendVariant/UDPSendVariantChannel/Send_RT_2015b ==
  SendData : Inport
  SendLen : Inport  Port=2
  Ground : Ground
  Send_RT_2015b : LopesDevelopmentLibrary/BlocksForInternalUse/LLC Communication/UDP_Blocks/Send_RT_2015b  ID=1  Send1=LopesParams.Communication.ipLLC_RT  Send2=port  Send3=-1  Send4=LopesParams.ts  udpID=0
  Dummy_out : Outport
  wires:
  SendLen/1 -> Send_RT_2015b/2
  SendData/1 -> Send_RT_2015b/1
  Ground/1 -> Dummy_out/1

== system LopesDevelopmentLibrary/GaitGeneration/CalculateBreaksCoefs/Calculate/Time1/CalculateStrideLength/GenerateReferencePoseLeftFront ==
  Phase : Inport
  BreaksCoefs : Inport  Port=2
  Parameters : Inport  Port=3
  CalculateCartesianPositions : LopesDevelopmentLibrary/BlocksForInternalUse/GaitGeneration/CalculateCartesianPositions
  CalculateReferenceGait : LopesDevelopmentLibrary/BlocksForInternalUse/GaitGeneration/CalculateReferenceGait
  Terminator{1..6} (6 alike) : Terminator
  true : Constant  Value=0
  CartesianPositions : Outport
  wires:
  CalculateCartesianPositions/2 -> Terminator6/1
  CalculateReferenceGait/4 -> Terminator5/1
  CalculateReferenceGait/3 -> Terminator4/1
  CalculateReferenceGait/2 -> Terminator3/1
  Phase/1 -> CalculateReferenceGait/1
  CalculateReferenceGait/1 -> CalculateCartesianPositions/2
  BreaksCoefs/1 -> CalculateReferenceGait/2
  Parameters/1 -> CalculateCartesianPositions/1, CalculateReferenceGait/3
  true/1 -> CalculateCartesianPositions/3
  CalculateReferenceGait/5 -> Terminator1/1
  CalculateReferenceGait/6 -> Terminator2/1
  CalculateCartesianPositions/1 -> CartesianPositions/1

== system LopesDevelopmentLibrary/GaitGeneration/CalculateBreaksCoefs/Calculate/Time1/CalculateStrideLength/GenerateReferencePoseRightFront ==
  Phase : Inport
  BreaksCoefs : Inport  Port=2
  Parameters : Inport  Port=3
  CalculateCartesianPositions : LopesDevelopmentLibrary/BlocksForInternalUse/GaitGeneration/CalculateCartesianPositions
  CalculateReferenceGait : LopesDevelopmentLibrary/BlocksForInternalUse/GaitGeneration/CalculateReferenceGait
  Terminator{1..6} (6 alike) : Terminator
  true : Constant  Value=0
  CartesianPositions : Outport
  wires:
  CalculateCartesianPositions/1 -> CartesianPositions/1
  CalculateReferenceGait/6 -> Terminator2/1
  CalculateReferenceGait/5 -> Terminator1/1
  true/1 -> CalculateCartesianPositions/3
  Parameters/1 -> CalculateReferenceGait/3, CalculateCartesianPositions/1
  BreaksCoefs/1 -> CalculateReferenceGait/2
  CalculateReferenceGait/1 -> CalculateCartesianPositions/2
  Phase/1 -> CalculateReferenceGait/1
  CalculateReferenceGait/2 -> Terminator3/1
  CalculateReferenceGait/3 -> Terminator4/1
  CalculateReferenceGait/4 -> Terminator5/1
  CalculateCartesianPositions/2 -> Terminator6/1

== system LopesDevelopmentLibrary/GaitGenerationExtra/CalculateBreaksCoefs/Calculate/Time1/CalculateStrideLength/GenerateReferencePoseLeftFront ==
  Phase : Inport
  BreaksCoefs : Inport  Port=2
  Parameters : Inport  Port=3
  CalculateCartesianPositions : LopesDevelopmentLibrary/BlocksForInternalUse/GaitGeneration/CalculateCartesianPositions
  CalculateReferenceGait : LopesDevelopmentLibrary/BlocksForInternalUse/GaitGeneration/CalculateReferenceGait
  Terminator{1..6} (6 alike) : Terminator
  true : Constant  Value=0
  CartesianPositions : Outport
  wires:
  CalculateCartesianPositions/2 -> Terminator6/1
  CalculateReferenceGait/4 -> Terminator5/1
  CalculateReferenceGait/3 -> Terminator4/1
  CalculateReferenceGait/2 -> Terminator3/1
  Phase/1 -> CalculateReferenceGait/1
  CalculateReferenceGait/1 -> CalculateCartesianPositions/2
  BreaksCoefs/1 -> CalculateReferenceGait/2
  Parameters/1 -> CalculateCartesianPositions/1, CalculateReferenceGait/3
  true/1 -> CalculateCartesianPositions/3
  CalculateReferenceGait/5 -> Terminator1/1
  CalculateReferenceGait/6 -> Terminator2/1
  CalculateCartesianPositions/1 -> CartesianPositions/1

== system LopesDevelopmentLibrary/GaitGenerationExtra/CalculateBreaksCoefs/Calculate/Time1/CalculateStrideLength/GenerateReferencePoseRightFront ==
  Phase : Inport
  BreaksCoefs : Inport  Port=2
  Parameters : Inport  Port=3
  CalculateCartesianPositions : LopesDevelopmentLibrary/BlocksForInternalUse/GaitGeneration/CalculateCartesianPositions
  CalculateReferenceGait : LopesDevelopmentLibrary/BlocksForInternalUse/GaitGeneration/CalculateReferenceGait
  Terminator{1..6} (6 alike) : Terminator
  true : Constant  Value=0
  CartesianPositions : Outport
  wires:
  CalculateCartesianPositions/1 -> CartesianPositions/1
  CalculateReferenceGait/6 -> Terminator2/1
  CalculateReferenceGait/5 -> Terminator1/1
  true/1 -> CalculateCartesianPositions/3
  Parameters/1 -> CalculateReferenceGait/3, CalculateCartesianPositions/1
  BreaksCoefs/1 -> CalculateReferenceGait/2
  CalculateReferenceGait/1 -> CalculateCartesianPositions/2
  Phase/1 -> CalculateReferenceGait/1
  CalculateReferenceGait/2 -> Terminator3/1
  CalculateReferenceGait/3 -> Terminator4/1
  CalculateReferenceGait/4 -> Terminator5/1
  CalculateCartesianPositions/2 -> Terminator6/1

== matlab function LopesDevelopmentLibrary/Robot control blocks/GeneralLopes/ShowStringInMatlabConsole ==
  data pre settings: description=Small string that is put in front of the received text.
  data: stringArray input; len input; pre input; enable input
function fcn(stringArray,len, pre, enable)
%#codegen
persistent t;
if isempty(t)
    t = 0;
end;
t = t+1;
    
coder.extrinsic('fprintf');
if (len~=0 && enable)
    fprintf('%6d: %s  (len = %d) - *%s*\n', t,char(pre'),len,char(stringArray(1:len).')); 
%    feval ('AddToGlobalXX',len);
end;

== matlab function LopesDevelopmentLibrary/StringFunctions/strlen ==
  data: s input; len output
function len = strlen(s)
%#codegen

% This function returns the length of the actual string, WITHOUT any
% trailing '\0's. So, the array  ['h','e','l','l','o',0,0,0,0] returns 5.
%
% s should be a uint8-array containing a string terminated with at least
% one '\0' character. The ASCII Encode block generates such an array
% (the array generated is fixed length, the first n bytes are the string,
% all other bytes are '\0'). 
%
% If the string does not have a trailing '\0' (in other words, if it is
% too large for its containing array), it returns the length of the array.

len = uint32(1);
maxlen = length(s);

while (len<= maxlen && s(len)~=0), 
    len = len + 1; 
end;
% Now len is the index of the first trailing '\0' (or maxlen+1);
% that is one more than the string length, so decrease by one:
len = len - 1;

== matlab function LopesDevelopmentLibrary/StringFunctions/concat ==
  data: s1 input; s1_len input; y output; s2 input; s2_len input; y_len output
function [y,y_len]= concat(s1,s1_len, s2, s2_len)
%#codegen

% Concatenates s1 and s2 into y, using a specified delimiter.
%
% s1 and s2 should be uint8-arrays containing a (possibly null-terminated) string.
% Usually, they will be a fixed-length array, holding the string in the
% first part; padded with zeros.
% s1_len and s2_len should be the actual string length (thus, the array
% uint8(['h','o','i',0,0,0,0]) has length 3. Use the strlen block for
% this.
%
% The result of this function is a fixed-length uint8-array, holding the
% string in the first part, padded with zeros, and the length of the
% resulting string (trailing zeros are not counted)
%
% If the resulting string would be too large to fit in the output array,
% it is truncated such that the output array is null-terminated and has
% maximum length.
%
% If s1_len> length(s1) (or similar with s2), the full length of the array
% will be taken as string.

%% Parameters
outputArrayLength = uint32(100); % The maximum string length is one less because of the trailing null-char
delimiter = uint8('; '); % Examples: uint8(';'), uint8('; ')
                        % Cannot be a non-empty string (if you don't want a delimiter, remove it from the Add() lines.


%% The work itself

i = uint32(1); % index within y
delimiter_len = length(delimiter);
y=zeros(outputArrayLength,1);

[y,i] = Add(s1, s1_len,              y, i, outputArrayLength);
[y,i] = Add(delimiter,delimiter_len, y, i, outputArrayLength);
[y,i] = Add(s2, s2_len,              y, i, outputArrayLength);

y_len = i-1;

%-------------------------------------------------
%% This subfunction actually adds the given string. If the output string
% is alrady 'full', nothing happens.
function [y, i] = Add(whichArray, stringLength, y, i, outputArrayLength)
nToCopy = min([length(whichArray),stringLength, outputArrayLength - i]);
if (nToCopy~=0),
    y(i:(i+nToCopy-1)) = whichArray(1:nToCopy);
    i = i + nToCopy;
end;

== matlab function LopesDevelopmentLibrary/StringFunctions/concat3 ==
  data: s1 input; s1_len input; y output; s2 input; s2_len input; y_len output; s3 input; s3_len input
function [y,y_len]= concat3(s1,s1_len, s2, s2_len,s3,s3_len)
%#codegen

% Concatenates s1 and s2, ... into y, using a specified delimiter.
%
% s1 and s2 should be uint8-arrays containing a (possibly null-terminated) string.
% Usually, they will be a fixed-length array, holding the string in the
% first part; padded with zeros.
% s1_len and s2_len should be the actual string length (thus, the array
% uint8(['h','o','i',0,0,0,0]) has length 3. Use the strlen block for
% this.
%
% The result of this function is a fixed-length uint8-array, holding the
% string in the first part, padded with zeros, and the length of the
% resulting string (trailing zeros are not counted)
%
% If the resulting string would be too large to fit in the output array,
% it is truncated such that the output array is null-terminated and has
% maximum length.
%
% If s1_len> length(s1) (or similar with s2), the full length of the array
% will be taken as string.

%% Parameters
outputArrayLength = uint32(100); % The maximum string length is one less because of the trailing null-char
delimiter = uint8(';'); % Examples: uint8(';'), uint8('; ')
                        % Cannot be a non-empty string (if you don't want a delimiter, remove it from the Add() lines.


%% The work itself

i = uint32(1); % index within y
delimiter_len = length(delimiter);
y=zeros(outputArrayLength,1);

[y,i] = Add(s1, s1_len,              y, i, outputArrayLength);
[y,i] = Add(delimiter,delimiter_len, y, i, outputArrayLength);
[y,i] = Add(s2, s2_len,              y, i, outputArrayLength);
[y,i] = Add(delimiter,delimiter_len, y, i, outputArrayLength);
[y,i] = Add(s3, s3_len,              y, i, outputArrayLength);

y_len = i-1;

%-------------------------------------------------
%% This subfunction actually adds the given string. If the output string
% is alrady 'full', nothing happens.
function [y, i] = Add(whichArray, stringLength, y, i, outputArrayLength)
nToCopy = min([length(whichArray),stringLength, outputArrayLength - i]);
if (nToCopy~=0),
    y(i:(i+nToCopy-1)) = whichArray(1:nToCopy);
    i = i + nToCopy;
end;
